simulink model "mix"  (R2022b)
settings: Solver=FixedStepAuto  StartTime=0.0  StopTime=10.0  FixedStep=0.1  RelTol=1e-3
values from neighbouring files (symbols this model uses):
  ModelInit_Att_qw = 0    [init.m]
  ModelInit_Att_qx = 1    [init.m]
  ModelInit_Att_qy = 0    [init.m]
  ModelInit_Att_qz = 0    [init.m]
  ModelInit_Pos_x = 0    [init.m]
  ModelInit_Pos_y = 0    [init.m]
  ModelInit_Pos_z = 0    [init.m]
  ModelParam_c_M = 1.779e-07*2    (= 3.558e-07)    [init.m]
  ModelParam_c_T = 1.105e-05    [init.m]
  ModelParam_d = 0.225    [init.m]
  ModelParam_g = 9.8    [init.m]
  ModelParam_I_xx = 0.0211    [init.m]
  ModelParam_I_yy = 0.0219    [init.m]
  ModelParam_I_zz = 0.0366    [init.m]
  ModelParam_J_RP = 0.0001287    [init.m]
  ModelParam_m = 1.4    [init.m]
settings Model: Creator=12854  LastModifiedBy=12854

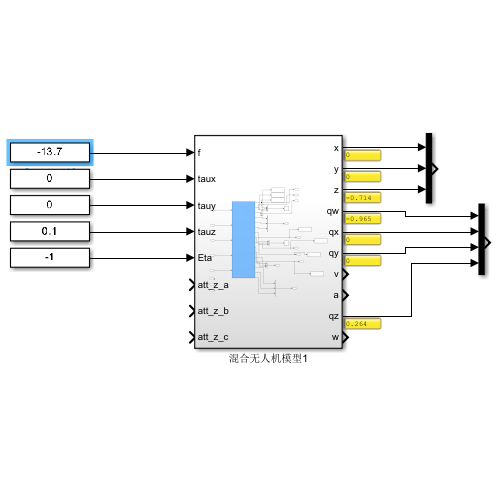
[thumbnail: Simulink's stored preview of the top-level diagram]
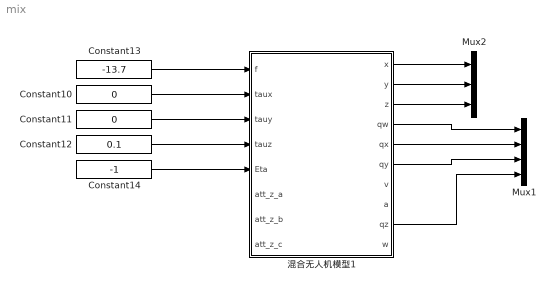
== system mix ==
  Constant10 : Constant  Value=0  SampleTime=0.1
  Constant11 : Constant  Value=0  SampleTime=0
  Constant12 : Constant  Value=0.1  SampleTime=0.1
  Constant13 : Constant  Value=-13.7  SampleTime=0.1
  Constant14 : Constant  Value=-1  SampleTime=0.1
  Mux1 : Mux
  Mux2 : Mux  Inputs=3
  混合无人机模型1 : Subsystem
  wires:
  Constant13/1 -> 混合无人机模型1/1(f)
  Constant14/1 -> 混合无人机模型1/5(Eta)
  Constant12/1 -> 混合无人机模型1/4(tauz)
  Constant10/1 -> 混合无人机模型1/2(taux)
  Constant11/1 -> 混合无人机模型1/3(tauy)
  混合无人机模型1/3(z) -> Mux2/3
  混合无人机模型1/2(y) -> Mux2/2
  混合无人机模型1/1(x) -> Mux2/1
  混合无人机模型1/4(qw) -> Mux1/1
  混合无人机模型1/5(qx) -> Mux1/2
  混合无人机模型1/6(qy) -> Mux1/3
  混合无人机模型1/9(qz) -> Mux1/4

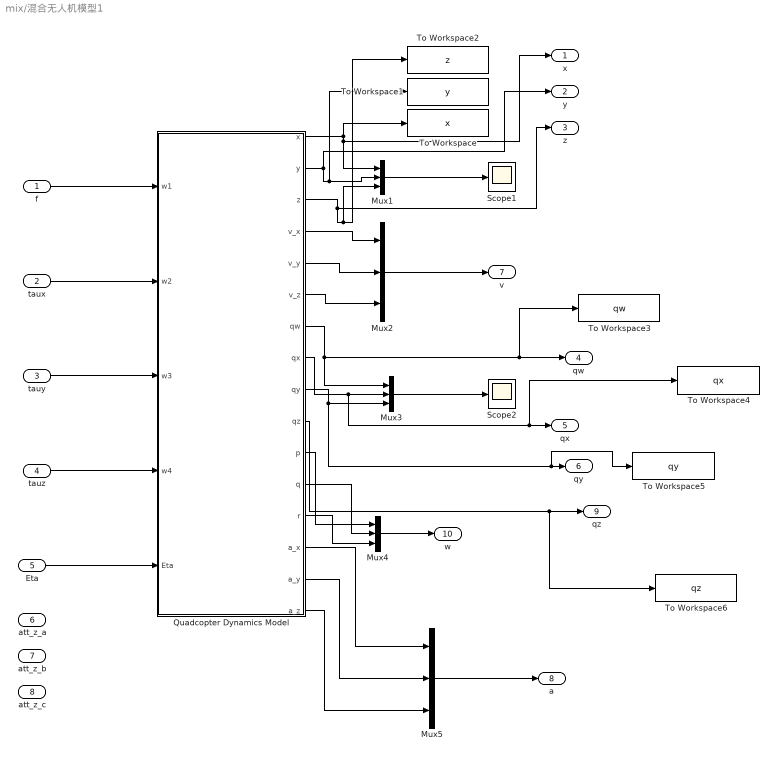
== system mix/混合无人机模型1 ==
  f : Inport  SampleTime=0.1
  taux : Inport  Port=2  SampleTime=0.1
  tauy : Inport  Port=3  SampleTime=0.1
  tauz : Inport  Port=4  SampleTime=0.1
  Eta : Inport  Port=5  SampleTime=0.1
  att_z_a : Inport  Port=6
  att_z_b : Inport  Port=7
  att_z_c : Inport  Port=8
  Mux{1..5} (5 alike) : Mux  Inputs=3
  Quadcopter Dynamics Model : Subsystem
  Scope1 : Scope
  Scope2 : Scope
  To Workspace : ToWorkspace  VariableName=x  SaveFormat=Timeseries  SampleTime=-1
  To Workspace1 : ToWorkspace  VariableName=y  SaveFormat=Timeseries  SampleTime=-1
  To Workspace2 : ToWorkspace  VariableName=z  SaveFormat=Timeseries  SampleTime=-1
  To Workspace3 : ToWorkspace  VariableName=qw  SaveFormat=Timeseries  SampleTime=-1
  To Workspace4 : ToWorkspace  VariableName=qx  SaveFormat=Timeseries  SampleTime=-1
  To Workspace5 : ToWorkspace  VariableName=qy  SaveFormat=Timeseries  SampleTime=-1
  To Workspace6 : ToWorkspace  VariableName=qz  SaveFormat=Timeseries  SampleTime=-1
  x : Outport
  y : Outport  Port=2
  z : Outport  Port=3
  qw : Outport  Port=4
  qx : Outport  Port=5
  qy : Outport  Port=6
  v : Outport  Port=7
  a : Outport  Port=8
  qz : Outport  Port=9
  w : Outport  Port=10
  wires:
  Mux3/1 -> Scope2/1
  Quadcopter Dynamics Model/2(y) -> To Workspace1/1, Mux1/2, y/1
  Quadcopter Dynamics Model/8(qx) -> To Workspace4/1, qx/1, Mux3/2
  Quadcopter Dynamics Model/5(v_y) -> Mux2/2
  Quadcopter Dynamics Model/1(x) -> Mux1/1, x/1, To Workspace/1
  Quadcopter Dynamics Model/6(v_z) -> Mux2/3
  Mux2/1 -> v/1
  Quadcopter Dynamics Model/13(r) -> Mux4/3
  Mux1/1 -> Scope1/1
  Quadcopter Dynamics Model/11(p) -> Mux4/1
  Quadcopter Dynamics Model/4(v_x) -> Mux2/1
  Quadcopter Dynamics Model/7(qw) -> Mux3/1, To Workspace3/1, qw/1
  Quadcopter Dynamics Model/3(z) -> To Workspace2/1, Mux1/3, z/1
  Quadcopter Dynamics Model/12(q) -> Mux4/2
  Quadcopter Dynamics Model/9(qy) -> To Workspace5/1, qy/1, Mux3/3
  f/1 -> Quadcopter Dynamics Model/1(w1)
  taux/1 -> Quadcopter Dynamics Model/2(w2)
  tauy/1 -> Quadcopter Dynamics Model/3(w3)
  tauz/1 -> Quadcopter Dynamics Model/4(w4)
  Quadcopter Dynamics Model/16(a_z) -> Mux5/3
  Quadcopter Dynamics Model/15(a_y) -> Mux5/2
  Quadcopter Dynamics Model/14(a_x) -> Mux5/1
  Mux5/1 -> a/1
  Quadcopter Dynamics Model/10(qz) -> To Workspace6/1, qz/1
  Eta/1 -> Quadcopter Dynamics Model/5(Eta)
  Mux4/1 -> w/1

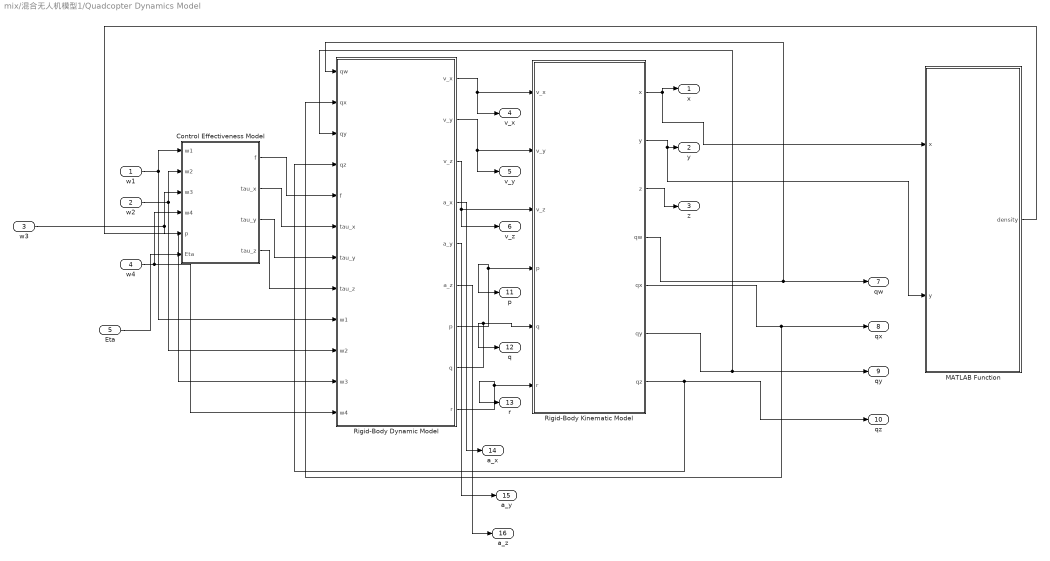
== system mix/混合无人机模型1/Quadcopter Dynamics Model ==
  w1 : Inport  SampleTime=0.1
  w2 : Inport  Port=2  SampleTime=0.1
  w3 : Inport  Port=3  SampleTime=0.1
  w4 : Inport  Port=4
  Eta : Inport  Port=5  SampleTime=0.1
  Control Effectiveness Model : Subsystem
  MATLAB Function : MATLAB Function  TreatAsAtomicUnit=on
  Rigid-Body Dynamic Model : Subsystem
  Rigid-Body Kinematic Model : Subsystem
  x : Outport  VectorParamsAs1DForOutWhenUnconnected=off
  y : Outport  Port=2  VectorParamsAs1DForOutWhenUnconnected=off
  z : Outport  Port=3  VectorParamsAs1DForOutWhenUnconnected=off
  v_x : Outport  Port=4  VectorParamsAs1DForOutWhenUnconnected=off
  v_y : Outport  Port=5  VectorParamsAs1DForOutWhenUnconnected=off
  v_z : Outport  Port=6  VectorParamsAs1DForOutWhenUnconnected=off
  qw : Outport  Port=7  VectorParamsAs1DForOutWhenUnconnected=off
  qx : Outport  Port=8  VectorParamsAs1DForOutWhenUnconnected=off
  qy : Outport  Port=9  VectorParamsAs1DForOutWhenUnconnected=off
  qz : Outport  Port=10  VectorParamsAs1DForOutWhenUnconnected=off
  p : Outport  Port=11  VectorParamsAs1DForOutWhenUnconnected=off
  q : Outport  Port=12  VectorParamsAs1DForOutWhenUnconnected=off
  r : Outport  Port=13  VectorParamsAs1DForOutWhenUnconnected=off
  a_x : Outport  Port=14  VectorParamsAs1DForOutWhenUnconnected=off
  a_y : Outport  Port=15  VectorParamsAs1DForOutWhenUnconnected=off
  a_z : Outport  Port=16  VectorParamsAs1DForOutWhenUnconnected=off
  wires:
  w1/1 -> Rigid-Body Dynamic Model/9(w1), Control Effectiveness Model/1(w1)
  w3/1 -> Rigid-Body Dynamic Model/11(w3), Control Effectiveness Model/3(w3)
  w4/1 -> Rigid-Body Dynamic Model/12(w4), Control Effectiveness Model/4(w4)
  w2/1 -> Control Effectiveness Model/2(w2), Rigid-Body Dynamic Model/10(w2)
  Rigid-Body Dynamic Model/7(p) -> p/1, Rigid-Body Kinematic Model/4(p)
  Rigid-Body Dynamic Model/9(r) -> r/1, Rigid-Body Kinematic Model/6(r)
  Control Effectiveness Model/2(tau_x) -> Rigid-Body Dynamic Model/6(tau_x)
  Rigid-Body Kinematic Model/1(x) -> x/1, MATLAB Function/1(x)
  Rigid-Body Dynamic Model/8(q) -> q/1, Rigid-Body Kinematic Model/5(q)
  Control Effectiveness Model/4(tau_z) -> Rigid-Body Dynamic Model/8(tau_z)
  Rigid-Body Kinematic Model/2(y) -> MATLAB Function/2(y), y/1
  Rigid-Body Kinematic Model/3(z) -> z/1
  Control Effectiveness Model/3(tau_y) -> Rigid-Body Dynamic Model/7(tau_y)
  Rigid-Body Kinematic Model/4(qw) -> Rigid-Body Dynamic Model/1(qw), qw/1
  Rigid-Body Kinematic Model/5(qx) -> Rigid-Body Dynamic Model/2(qx), qx/1
  Rigid-Body Kinematic Model/6(qy) -> Rigid-Body Dynamic Model/3(qy), qy/1
  MATLAB Function/1(density) -> Control Effectiveness Model/5(p)
  Rigid-Body Dynamic Model/4(a_x) -> a_x/1
  Rigid-Body Dynamic Model/5(a_y) -> a_y/1
  Rigid-Body Dynamic Model/6(a_z) -> a_z/1
  Rigid-Body Dynamic Model/1(v_x) -> Rigid-Body Kinematic Model/1(v_x), v_x/1
  Rigid-Body Dynamic Model/2(v_y) -> Rigid-Body Kinematic Model/2(v_y), v_y/1
  Rigid-Body Dynamic Model/3(v_z) -> Rigid-Body Kinematic Model/3(v_z), v_z/1
  Control Effectiveness Model/1(f) -> Rigid-Body Dynamic Model/5(f)
  Rigid-Body Kinematic Model/7(qz) -> Rigid-Body Dynamic Model/4(qz), qz/1
  Eta/1 -> Control Effectiveness Model/6(Eta)

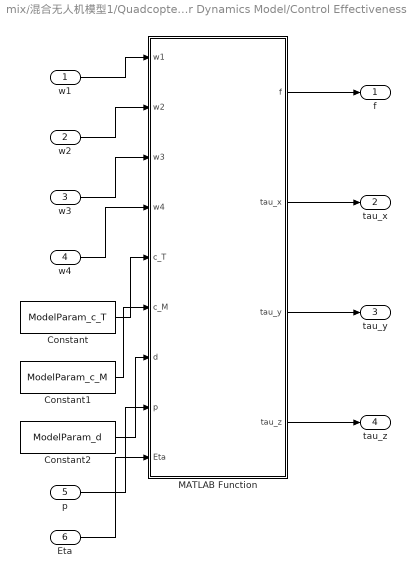
== system mix/混合无人机模型1/Quadcopter Dynamics Model/Control Effectiveness Model ==
  w1 : Inport
  w2 : Inport  Port=2
  w3 : Inport  Port=3
  w4 : Inport  Port=4
  p : Inport  Port=5
  Eta : Inport  Port=6
  Constant : Constant  Value=ModelParam_c_T
  Constant1 : Constant  Value=ModelParam_c_M
  Constant2 : Constant  Value=ModelParam_d
  MATLAB Function : MATLAB Function  TreatAsAtomicUnit=on  SystemSampleTime=0.1
  f : Outport  VectorParamsAs1DForOutWhenUnconnected=off
  tau_x : Outport  Port=2  VectorParamsAs1DForOutWhenUnconnected=off
  tau_y : Outport  Port=3  VectorParamsAs1DForOutWhenUnconnected=off
  tau_z : Outport  Port=4  VectorParamsAs1DForOutWhenUnconnected=off
  wires:
  Constant1/1 -> MATLAB Function/6(c_M)
  Constant/1 -> MATLAB Function/5(c_T)
  MATLAB Function/3(tau_y) -> tau_y/1
  MATLAB Function/1(f) -> f/1
  Constant2/1 -> MATLAB Function/7(d)
  MATLAB Function/4(tau_z) -> tau_z/1
  w3/1 -> MATLAB Function/3(w3)
  w1/1 -> MATLAB Function/1(w1)
  w4/1 -> MATLAB Function/4(w4)
  MATLAB Function/2(tau_x) -> tau_x/1
  w2/1 -> MATLAB Function/2(w2)
  p/1 -> MATLAB Function/8(p)
  Eta/1 -> MATLAB Function/9(Eta)

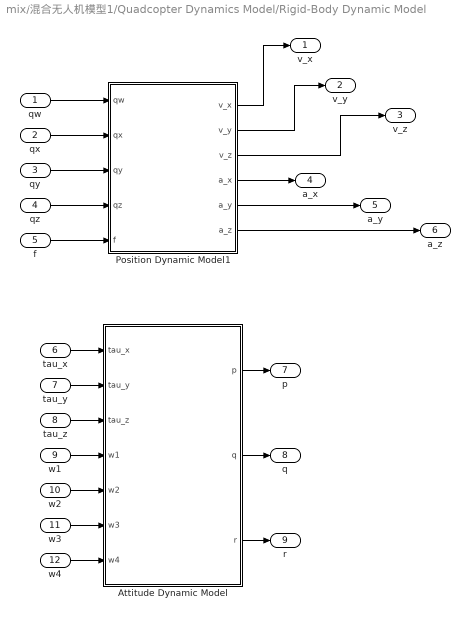
== system mix/混合无人机模型1/Quadcopter Dynamics Model/Rigid-Body Dynamic Model ==
  qw : Inport
  qx : Inport  Port=2
  qy : Inport  Port=3
  qz : Inport  Port=4
  f : Inport  Port=5
  tau_x : Inport  Port=6
  tau_y : Inport  Port=7
  tau_z : Inport  Port=8
  w1 : Inport  Port=9
  w2 : Inport  Port=10
  w3 : Inport  Port=11
  w4 : Inport  Port=12
  Attitude Dynamic Model : Subsystem
  Position Dynamic Model1 : Subsystem
  v_x : Outport  VectorParamsAs1DForOutWhenUnconnected=off
  v_y : Outport  Port=2  VectorParamsAs1DForOutWhenUnconnected=off
  v_z : Outport  Port=3  VectorParamsAs1DForOutWhenUnconnected=off
  a_x : Outport  Port=4  VectorParamsAs1DForOutWhenUnconnected=off
  a_y : Outport  Port=5  VectorParamsAs1DForOutWhenUnconnected=off
  a_z : Outport  Port=6  VectorParamsAs1DForOutWhenUnconnected=off
  p : Outport  Port=7  VectorParamsAs1DForOutWhenUnconnected=off
  q : Outport  Port=8  VectorParamsAs1DForOutWhenUnconnected=off
  r : Outport  Port=9  VectorParamsAs1DForOutWhenUnconnected=off
  wires:
  w3/1 -> Attitude Dynamic Model/6(w3)
  w1/1 -> Attitude Dynamic Model/4(w1)
  tau_x/1 -> Attitude Dynamic Model/1(tau_x)
  w2/1 -> Attitude Dynamic Model/5(w2)
  Attitude Dynamic Model/1(p) -> p/1
  w4/1 -> Attitude Dynamic Model/7(w4)
  Attitude Dynamic Model/2(q) -> q/1
  tau_y/1 -> Attitude Dynamic Model/2(tau_y)
  tau_z/1 -> Attitude Dynamic Model/3(tau_z)
  Attitude Dynamic Model/3(r) -> r/1
  qw/1 -> Position Dynamic Model1/1(qw)
  qx/1 -> Position Dynamic Model1/2(qx)
  qy/1 -> Position Dynamic Model1/3(qy)
  qz/1 -> Position Dynamic Model1/4(qz)
  f/1 -> Position Dynamic Model1/5(f)
  Position Dynamic Model1/1(v_x) -> v_x/1
  Position Dynamic Model1/2(v_y) -> v_y/1
  Position Dynamic Model1/3(v_z) -> v_z/1
  Position Dynamic Model1/4(a_x) -> a_x/1
  Position Dynamic Model1/5(a_y) -> a_y/1
  Position Dynamic Model1/6(a_z) -> a_z/1

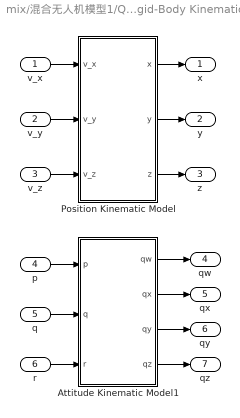
== system mix/混合无人机模型1/Quadcopter Dynamics Model/Rigid-Body Kinematic Model ==
  v_x : Inport
  v_y : Inport  Port=2
  v_z : Inport  Port=3
  p : Inport  Port=4
  q : Inport  Port=5
  r : Inport  Port=6
  Attitude Kinematic Model1 : Subsystem
  Position Kinematic Model : Subsystem
  x : Outport  VectorParamsAs1DForOutWhenUnconnected=off
  y : Outport  Port=2  VectorParamsAs1DForOutWhenUnconnected=off
  z : Outport  Port=3  VectorParamsAs1DForOutWhenUnconnected=off
  qw : Outport  Port=4  VectorParamsAs1DForOutWhenUnconnected=off
  qx : Outport  Port=5  VectorParamsAs1DForOutWhenUnconnected=off
  qy : Outport  Port=6  VectorParamsAs1DForOutWhenUnconnected=off
  qz : Outport  Port=7  VectorParamsAs1DForOutWhenUnconnected=off
  wires:
  v_x/1 -> Position Kinematic Model/1(v_x)
  v_y/1 -> Position Kinematic Model/2(v_y)
  r/1 -> Attitude Kinematic Model1/3(r)
  p/1 -> Attitude Kinematic Model1/1(p)
  v_z/1 -> Position Kinematic Model/3(v_z)
  Position Kinematic Model/1(x) -> x/1
  Position Kinematic Model/2(y) -> y/1
  q/1 -> Attitude Kinematic Model1/2(q)
  Position Kinematic Model/3(z) -> z/1
  Attitude Kinematic Model1/2(qx) -> qx/1
  Attitude Kinematic Model1/1(qw) -> qw/1
  Attitude Kinematic Model1/3(qy) -> qy/1
  Attitude Kinematic Model1/4(qz) -> qz/1

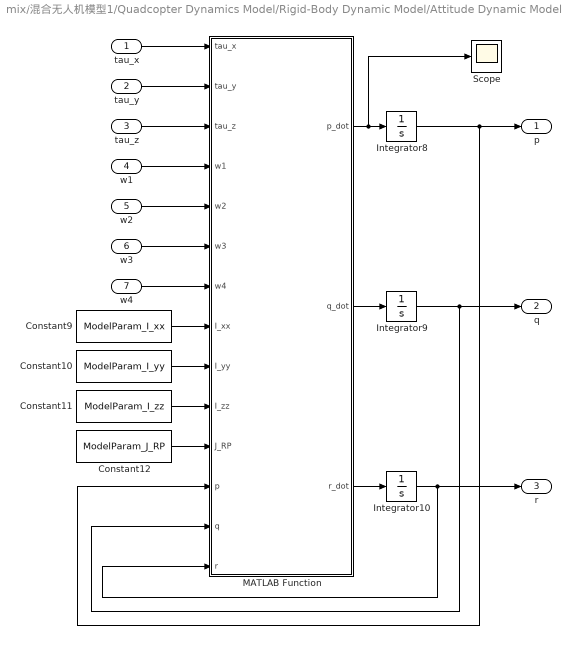
== system mix/混合无人机模型1/Quadcopter Dynamics Model/Rigid-Body Dynamic Model/Attitude Dynamic Model ==
  tau_x : Inport
  tau_y : Inport  Port=2
  tau_z : Inport  Port=3
  w1 : Inport  Port=4
  w2 : Inport  Port=5
  w3 : Inport  Port=6
  w4 : Inport  Port=7
  Constant10 : Constant  Value=ModelParam_I_yy
  Constant11 : Constant  Value=ModelParam_I_zz
  Constant12 : Constant  Value=ModelParam_J_RP
  Constant9 : Constant  Value=ModelParam_I_xx
  Integrator10 : Integrator
  Integrator8 : Integrator
  Integrator9 : Integrator
  MATLAB Function : MATLAB Function  TreatAsAtomicUnit=on  SystemSampleTime=0.1
  Scope : Scope
  p : Outport  VectorParamsAs1DForOutWhenUnconnected=off
  q : Outport  Port=2  VectorParamsAs1DForOutWhenUnconnected=off
  r : Outport  Port=3  VectorParamsAs1DForOutWhenUnconnected=off
  wires:
  Constant9/1 -> MATLAB Function/8(I_xx)
  tau_z/1 -> MATLAB Function/3(tau_z)
  Integrator10/1 -> r/1, MATLAB Function/14(r)
  Constant12/1 -> MATLAB Function/11(J_RP)
  Integrator9/1 -> q/1, MATLAB Function/13(q)
  Constant10/1 -> MATLAB Function/9(I_yy)
  MATLAB Function/3(r_dot) -> Integrator10/1
  MATLAB Function/1(p_dot) -> Scope/1, Integrator8/1
  Integrator8/1 -> p/1, MATLAB Function/12(p)
  tau_y/1 -> MATLAB Function/2(tau_y)
  MATLAB Function/2(q_dot) -> Integrator9/1
  Constant11/1 -> MATLAB Function/10(I_zz)
  w1/1 -> MATLAB Function/4(w1)
  tau_x/1 -> MATLAB Function/1(tau_x)
  w2/1 -> MATLAB Function/5(w2)
  w3/1 -> MATLAB Function/6(w3)
  w4/1 -> MATLAB Function/7(w4)

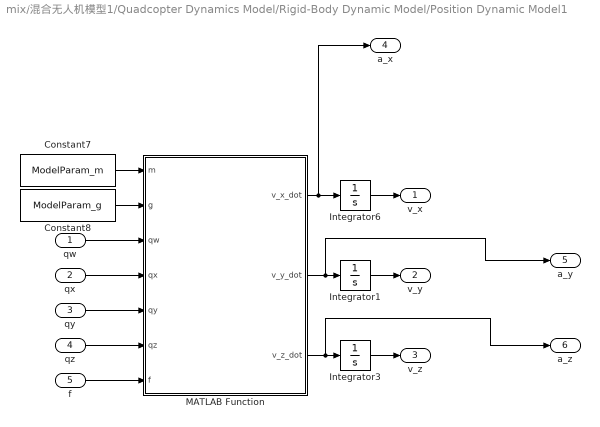
== system mix/混合无人机模型1/Quadcopter Dynamics Model/Rigid-Body Dynamic Model/Position Dynamic Model1 ==
  qw : Inport  SampleTime=0.1
  qx : Inport  Port=2
  qy : Inport  Port=3
  qz : Inport  Port=4
  f : Inport  Port=5
  Constant7 : Constant  Value=ModelParam_m  SampleTime=0.1
  Constant8 : Constant  Value=ModelParam_g  SampleTime=0.1
  Integrator1 : Integrator
  Integrator3 : Integrator
  Integrator6 : Integrator
  MATLAB Function : MATLAB Function  TreatAsAtomicUnit=on  SystemSampleTime=0.1
  v_x : Outport  VectorParamsAs1DForOutWhenUnconnected=off
  v_y : Outport  Port=2  VectorParamsAs1DForOutWhenUnconnected=off
  v_z : Outport  Port=3  VectorParamsAs1DForOutWhenUnconnected=off
  a_x : Outport  Port=4  VectorParamsAs1DForOutWhenUnconnected=off
  a_y : Outport  Port=5  VectorParamsAs1DForOutWhenUnconnected=off
  a_z : Outport  Port=6  VectorParamsAs1DForOutWhenUnconnected=off
  wires:
  Constant8/1 -> MATLAB Function/2(g)
  MATLAB Function/1(v_x_dot) -> a_x/1, Integrator6/1
  MATLAB Function/2(v_y_dot) -> a_y/1, Integrator1/1
  qx/1 -> MATLAB Function/4(qx)
  Constant7/1 -> MATLAB Function/1(m)
  MATLAB Function/3(v_z_dot) -> a_z/1, Integrator3/1
  qw/1 -> MATLAB Function/3(qw)
  f/1 -> MATLAB Function/7(f)
  qy/1 -> MATLAB Function/5(qy)
  Integrator6/1 -> v_x/1
  Integrator1/1 -> v_y/1
  Integrator3/1 -> v_z/1
  qz/1 -> MATLAB Function/6(qz)

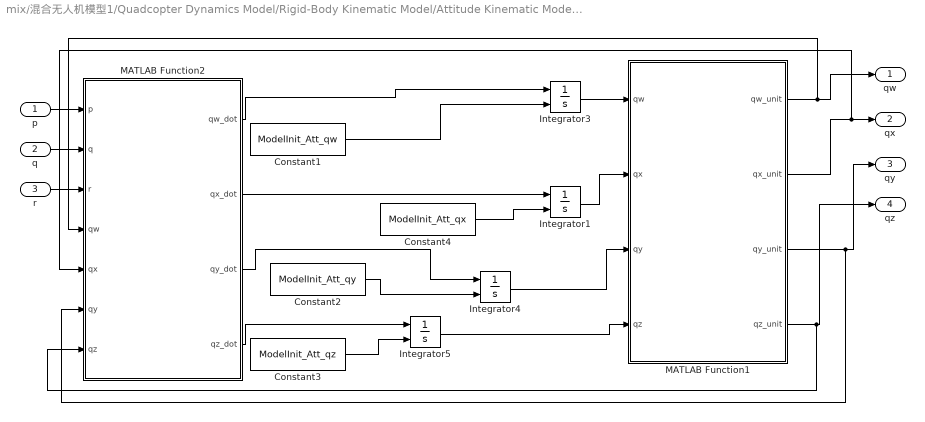
== system mix/混合无人机模型1/Quadcopter Dynamics Model/Rigid-Body Kinematic Model/Attitude Kinematic Model1 ==
  p : Inport
  q : Inport  Port=2
  r : Inport  Port=3
  Constant1 : Constant  Value=ModelInit_Att_qw
  Constant2 : Constant  Value=ModelInit_Att_qy
  Constant3 : Constant  Value=ModelInit_Att_qz
  Constant4 : Constant  Value=ModelInit_Att_qx
  Integrator{1,3..5} (4 alike) : Integrator  InitialConditionSource=external
  MATLAB Function1 : MATLAB Function  TreatAsAtomicUnit=on
  MATLAB Function2 : MATLAB Function  TreatAsAtomicUnit=on
  qw : Outport  VectorParamsAs1DForOutWhenUnconnected=off
  qx : Outport  Port=2  VectorParamsAs1DForOutWhenUnconnected=off
  qy : Outport  Port=3  VectorParamsAs1DForOutWhenUnconnected=off
  qz : Outport  Port=4  VectorParamsAs1DForOutWhenUnconnected=off
  wires:
  r/1 -> MATLAB Function2/3(r)
  MATLAB Function2/1(qw_dot) -> Integrator3/1
  q/1 -> MATLAB Function2/2(q)
  p/1 -> MATLAB Function2/1(p)
  Constant1/1 -> Integrator3/2
  Constant2/1 -> Integrator4/2
  Constant3/1 -> Integrator5/2
  MATLAB Function2/2(qx_dot) -> Integrator1/1
  Constant4/1 -> Integrator1/2
  MATLAB Function2/3(qy_dot) -> Integrator4/1
  MATLAB Function2/4(qz_dot) -> Integrator5/1
  Integrator3/1 -> MATLAB Function1/1(qw)
  Integrator1/1 -> MATLAB Function1/2(qx)
  Integrator4/1 -> MATLAB Function1/3(qy)
  Integrator5/1 -> MATLAB Function1/4(qz)
  MATLAB Function1/1(qw_unit) -> MATLAB Function2/4(qw), qw/1
  MATLAB Function1/2(qx_unit) -> MATLAB Function2/5(qx), qx/1
  MATLAB Function1/3(qy_unit) -> MATLAB Function2/6(qy), qy/1
  MATLAB Function1/4(qz_unit) -> MATLAB Function2/7(qz), qz/1

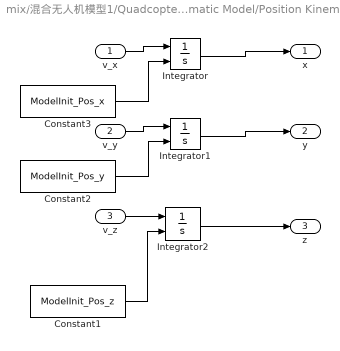
== system mix/混合无人机模型1/Quadcopter Dynamics Model/Rigid-Body Kinematic Model/Position Kinematic Model ==
  v_x : Inport
  v_y : Inport  Port=2
  v_z : Inport  Port=3
  Constant1 : Constant  Value=ModelInit_Pos_z
  Constant2 : Constant  Value=ModelInit_Pos_y
  Constant3 : Constant  Value=ModelInit_Pos_x
  Integrator : Integrator  InitialConditionSource=external
  Integrator1 : Integrator  InitialConditionSource=external
  Integrator2 : Integrator  InitialConditionSource=external
  x : Outport  VectorParamsAs1DForOutWhenUnconnected=off
  y : Outport  Port=2  VectorParamsAs1DForOutWhenUnconnected=off
  z : Outport  Port=3  VectorParamsAs1DForOutWhenUnconnected=off
  wires:
  v_z/1 -> Integrator2/1
  Integrator1/1 -> y/1
  Integrator/1 -> x/1
  Constant1/1 -> Integrator2/2
  Integrator2/1 -> z/1
  v_x/1 -> Integrator/1
  v_y/1 -> Integrator1/1
  Constant2/1 -> Integrator1/2
  Constant3/1 -> Integrator/2

== matlab function mix/混合无人机模型1/Quadcopter Dynamics Model/Control Effectiveness Model/MATLAB Function ==
  data: w1 input; f output; w2 input; w3 input; w4 input; c_T input; c_M input; d input; tau_x output; tau_y output; tau_z output; p input; Eta input
function [f, tau_x, tau_y, tau_z] = fcn(w1, w2, w3, w4, c_T, c_M, d, p, Eta)
% 函数描述
% 1.作用：本函数用来计算螺旋桨旋转产生的总拉力和反扭力矩。
% 2.函数输入：
%   wi：四个螺旋桨的转速(rad/s)，可以为正或负
%   c_T：螺旋桨拉力系数和外面的converter的CT不同，已经经过换算就等于KF
%   c_M：螺旋桨转矩系数= KM
%   d：机体中心和任一电机的距离(m)
% 3.函数输出：
%   f：螺旋桨拉力（机体轴）
%   tau_x：x轴反扭力矩（机体轴）
%   tau_y：y轴反扭力矩（机体轴）
%   tau_z：z轴反扭力矩（机体轴）
% 4.四旋翼构型为"+”型，螺旋桨序号如下所示：
%            y
%            2↑
%            |
%        3↓—— —— 1↓   x
%            |
%            4↑
f=w1;tau_x=w2;tau_y=w3;tau_z=w4;
if Eta == 1
    f=w1;tau_x=w2;tau_y=w3;tau_z=w4;
end

if Eta == -1
    f=-w1;tau_x=w2;tau_y=w3;tau_z=w4;
end

== matlab function mix/混合无人机模型1/Quadcopter Dynamics Model/MATLAB Function ==
  data: x input; density output; y input
function density = air_density(x, y)
    % 定义火坑的中心位置
    center_x = 10;
    center_y = 10;

    % 定义火坑的半径
    radius = 0.00001;

    % 定义火坑中心的空气密度为1.078 kg/m³
    density_center = 1.078;

    % 定义火坑边缘的空气密度为日常密度值
    density_edge = 1.225;

    % 计算无人机到火坑中心的距离
    r = sqrt((x - center_x)^2 + (y - center_y)^2);

    % 定义高斯函数的标准差
    sigma = radius / 3;
    
    % 使用高斯函数计算空气密度
    density = density_edge + (density_center - density_edge) * exp(-(r.^2) / (2 * sigma^2));


    density = density/1.225;
end

== matlab function mix/混合无人机模型1/Quadcopter Dynamics Model/Rigid-Body Dynamic Model/Attitude Dynamic Model/MATLAB Function ==
  data: tau_x input; p_dot output; tau_y input; tau_z input; w1 input; w2 input; w3 input; w4 input; I_xx input; I_yy input; I_zz input; J_RP input; p input; q input; r input; q_dot output; r_dot output
function [p_dot, q_dot, r_dot] = fcn(tau_x, tau_y, tau_z, w1, w2, w3, w4, I_xx, I_yy, I_zz, J_RP, p, q, r)
% 函数描述
% 1.作用：本函数为四旋翼的姿态动力学微分方程组，通过四旋翼所受力矩和螺旋
%         桨转速计算得到四旋翼的机体角速度
% 2.函数输入：
%   wi：四个螺旋桨的转速(rad/s)
%   tau_x：x轴反扭力矩（机体轴）(N·m)
%   tau_y：y轴反扭力矩（机体轴）(N·m)
%   tau_z：z轴反扭力矩（机体轴）(N·m)
%   I_xx：四旋翼x轴转动惯量(kg·m^2)
%   I_yy：四旋翼y轴转动惯量(kg·m^2)
%   I_zz：四旋翼z轴转动惯量(kg·m^2)
%   J_RP：整个电机转子和螺旋桨绕转轴的总转动惯量(kg·m^2)
%   p：四旋翼x轴角速度（机体轴)(rad/s)
%   q：四旋翼y轴角速度（机体轴)(rad/s)
%   r：四旋翼z轴角速度（机体轴)(rad/s)
% 3.函数输出：
%   p_dot：四旋翼x轴角加速度（机体轴)
%   q_dot：四旋翼y轴角加速度（机体轴)
%   r_dot：四旋翼z轴角加速度（机体轴)
% 4.四旋翼构型为“X”型，螺旋桨序号如下所示：
%            y
%            2↑
%            |
%        3↓—— —— 1↓   x
%            |
%            4↑
%   其中，↑表示螺旋桨逆时针旋转；↓表示螺旋桨顺时针旋转。


p_dot = (1/I_xx) * (tau_x + q * r * (I_yy - I_zz) );
q_dot = (1/I_yy) * (tau_y + p * r * (I_zz - I_xx) );
r_dot = (1/I_zz) * (tau_z + p * q * (I_xx - I_yy) );
end

== matlab function mix/混合无人机模型1/Quadcopter Dynamics Model/Rigid-Body Dynamic Model/Position Dynamic Model1/MATLAB Function ==
  data: m input; g input; qw input; qx input; qy input; qz input; f input; v_x_dot output; v_y_dot output; v_z_dot output
function [v_x_dot, v_y_dot, v_z_dot] = fcn(m, g, qw, qx, qy, qz, f)
% 函数描述
% 1.作用：本函数为四旋翼的位置动力学微分方程组，通过四旋翼所受拉力、姿态角
%         计算得到四旋翼飞行器的加速度
% 2.函数输入：
%   m：四旋翼飞行器质量(kg)
%   g：重力加速度(m/s^2)
%   qw：四元数1号位
%   qx：四元数2号位
%   qy：四元数3号位
%   qz：四元数4号位
%   f：螺旋桨产生的总拉力(N)
% 3.函数输出：
%   v_x_dot：地球坐标系下沿x轴的速度的导数
%   v_y_dot：地球坐标系下沿y轴的速度的导数
%   v_z_dot：地球坐标系下沿z轴的速度的导数
% 4.四旋翼构型为"+”型，螺旋桨序号如下所示：
%            y
%            2↑
%            |
%        3↓—— —— 1↓   x
%            |
%            4↑
%   其中，↑表示螺旋桨逆时针旋转；↓表示螺旋桨顺时针旋转。
% 计算旋转矩阵 R
R11 = 1 - 2*qy^2 - 2*qz^2;
R12 = 2*qx*qy - 2*qz*qw;
R13 = 2*qx*qz + 2*qy*qw
R21 = 2*qx*qy + 2*qz*qw;
R22 = 1 - 2*qx^2 - 2*qz^2;
R23 = 2*qy*qz - 2*qx*qw
R31 = 2*qx*qz - 2*qy*qw;
R32 = 2*qy*qz + 2*qx*qw;
R33 = 1 - 2*qx^2 - 2*qy^2

v_x_dot = f * (1/m) * (R13)
v_y_dot = f * (1/m) * (R23)
v_z_dot = f * (1/m) * R33 - g
end

== matlab function mix/混合无人机模型1/Quadcopter Dynamics Model/Rigid-Body Kinematic Model/Attitude Kinematic Model1/MATLAB Function1 ==
  data: qw_unit output; qw input; qx input; qy input; qz input; qx_unit output; qy_unit output; qz_unit output
function [qw_unit, qx_unit, qy_unit, qz_unit] = normalize_quaternion(qw, qx, qy, qz)
    % 计算四元数的模
    norm_q = sqrt(qw^2 + qx^2 + qy^2 + qz^2);
    
    % 检查模是否为零，避免除以零的错误
    if norm_q == 0
        error('Zero norm quaternion cannot be normalized.');
    end

    % 单位化四元数
    qw_unit = qw / norm_q;
    qx_unit = qx / norm_q;
    qy_unit = qy / norm_q;
    qz_unit = qz / norm_q;
end

== matlab function mix/混合无人机模型1/Quadcopter Dynamics Model/Rigid-Body Kinematic Model/Attitude Kinematic Model1/MATLAB Function2 ==
  data: p input; qw_dot output; q input; r input; qw input; qx input; qy input; qz input; qx_dot output; qy_dot output; qz_dot output
function [qw_dot, qx_dot, qy_dot, qz_dot] = updateQuaternion(p, q, r, qw, qx, qy, qz)
    % updateQuaternion 更新无人机的姿态四元数
    % 输入:
    %   q - 当前姿态四元数，形式为 [qw, qx, qy, qz]
    %   omega - 三轴角速度，形式为 [omega_x, omega_y, omega_z]
    %   dt - 时间步长

    % 将角速度转换为四元数形式
    q_current = [qw, qx, qy, qz];
    omega_q = [0, p, q, r];
    
    % 计算四元数的导数
    q_dot = 0.5 * quatmultiply(omega_q, q_current);
    qw_dot = q_dot(1);
    qx_dot = q_dot(2);
    qy_dot = q_dot(3);
    qz_dot = q_dot(4);
end
